simulink model "W03_Pendulum_NonlinVsLin"  (R2024b)
settings: Solver=ode45  StartTime=0.0  StopTime=t_end  MaxStep=0.01  RelTol=1e-3
PreLoadFcn:
  | % W03_Pendulum_NonlinVsLin 기본 파라미터 (모델을 열 때 자동 실행)
  | % 이미 워크스페이스에 값이 있으면 그대로 두고, 없을 때만 채웁니다.
  | defs = { 'm',0.5 ; 'l',0.3 ; 'b',0 ; 'g',9.81 ;
  |          'u_torque',0 ; 'theta0',pi/3 ; 't_end',10 };
  | for ii = 1:size(defs,1)
  |     if ~evalin('base', sprintf('exist(''%s'',''var'')', defs{ii,1}))
  |         assignin('base', defs{ii,1}, defs{ii,2});
  |     end
  | end
  | clear defs ii
values from neighbouring files (symbols this model uses):
  b = 0.2    [W03_02_state_space.m]    (also in W03_04_run_simulink.m = p.b; W03_05_linearize_verify.m = 0.15)
  g = p.g    [W03_04_run_simulink.m]    (also in W03_05_linearize_verify.m = 9.81)
  l = p.l    [W03_04_run_simulink.m]    (also in W03_05_linearize_verify.m = 0.3)
  m = 1    [W03_02_state_space.m]    (also in W03_04_run_simulink.m = p.m; W03_05_linearize_verify.m = 0.5)
  theta0 = deg2rad(angle_list(i))    [W03_04_run_simulink.m]    (also in W03_05_linearize_verify.m = 0)
  u_torque = 0    [W03_04_run_simulink.m]    (also in W03_05_linearize_verify.m)
settings Model: Creator=admin  LastModifiedBy=admin

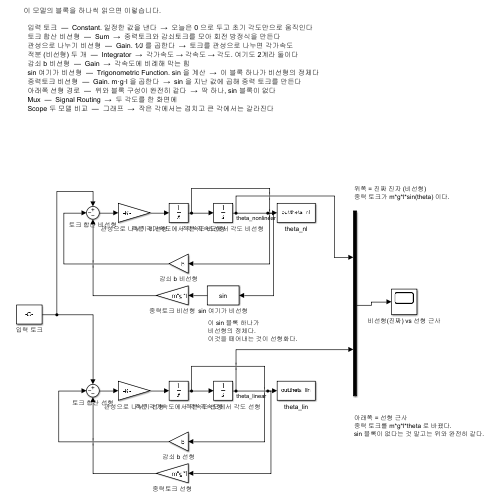
[thumbnail: Simulink's stored preview of the top-level diagram]
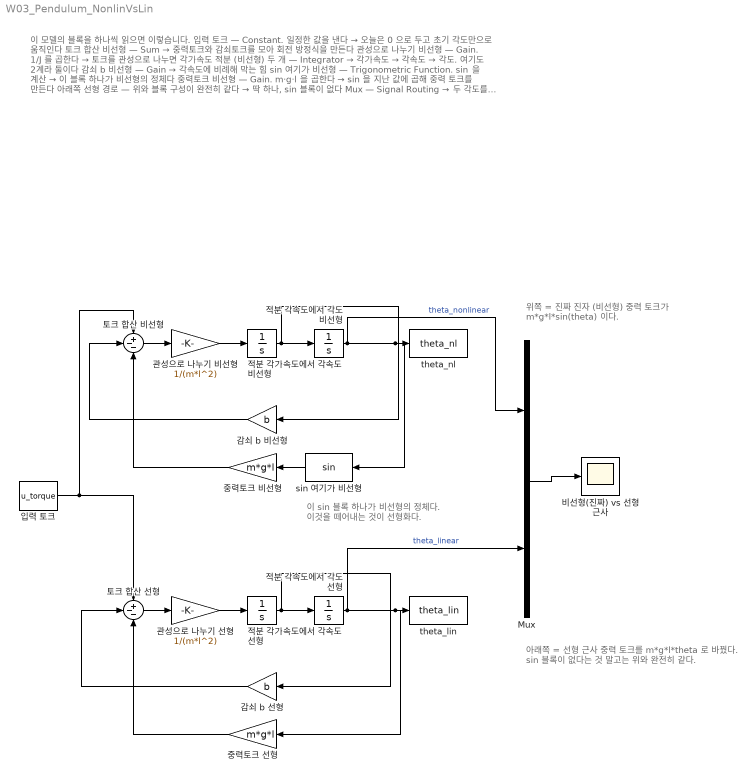
== system W03_Pendulum_NonlinVsLin ==
  note: 위쪽 = 진짜 진자 (비선형)
      | 중력 토크가 m*g*l*sin(theta) 이다.
  note: 아래쪽 = 선형 근사
      | 중력 토크를 m*g*l*theta 로 바꿨다.
      | sin 블록이 없다는 것 말고는 위와 완전히 같다.
  note: 이 sin 블록 하나가
      | 비선형의 정체다.
      | 이것을 떼어내는 것이 선형화다.
  note: 이 모델의 블록을 하나씩 읽으면 이렇습니다.
      |
      |   입력 토크  —  Constant. 일정한 값을 낸다  →  오늘은 0 으로 두고 초기 각도만으로 움직인다
      |   토크 합산 비선형  —  Sum  →  중력토크와 감쇠토크를 모아 회전 방정식을 만든다
      |   관성으로 나누기 비선형  —  Gain. 1∕J 를 곱한다  →  토크를 관성으로 나누면 각가속도
      |   적분 (비선형) 두 개  —  Integrator  →  각가속도 → 각속도 → 각도. 여기도 2계라 둘이다
      |   감쇠 b 비선형  —  Gain  →  각속도에 비례해 막는 힘
      |   sin 여기가 비선형  —  Trigonometric Function. sin 을 계산  →  이 블록 하나가 비선형의 정체다
      |   중력토크 비선형  —  Gain. m·g·l 을 곱한다  →  sin 을 지난 값에 곱해 중력 토크를 만든다
      |   아래쪽 선형 경로  —  위와 블록 구성이 완전히 같다  →  딱 하나, sin 블록이 없다
      |   Mux  —  Signal Routing  →  두 각도를 한 화면에
      |   Scope 두 모델 비교  —  그래프  →  작은 각에서는 겹치고 큰 각에서는 갈라진다
  Mux : Mux  Inputs=2
  sin 여기가 비선형 : Trigonometry
  theta_lin : ToWorkspace  VariableName=theta_lin  SaveFormat=Timeseries  SampleTime=-1
  theta_nl : ToWorkspace  VariableName=theta_nl  SaveFormat=Timeseries  SampleTime=-1
  감쇠 b 비선형 : Gain  Gain=b
  감쇠 b 선형 : Gain  Gain=b
  관성으로 나누기 비선형 : Gain  Gain=1/(m*l^2)
  관성으로 나누기 선형 : Gain  Gain=1/(m*l^2)
  비선형(진짜) vs 선형 근사 : Scope
  입력 토크 : Constant  Value=u_torque
  적분 각가속도에서 각속도 비선형 : Integrator
  적분 각가속도에서 각속도 선형 : Integrator
  적분 각속도에서 각도 비선형 : Integrator  InitialCondition=theta0
  적분 각속도에서 각도 선형 : Integrator  InitialCondition=theta0
  중력토크 비선형 : Gain  Gain=m*g*l
  중력토크 선형 : Gain  Gain=m*g*l
  토크 합산 비선형 : Sum  Inputs=+--
  토크 합산 선형 : Sum  Inputs=+--
  wires:
  입력 토크/1 -> 토크 합산 비선형/1, 토크 합산 선형/1
  토크 합산 비선형/1 -> 관성으로 나누기 비선형/1
  관성으로 나누기 비선형/1 -> 적분 각가속도에서 각속도 비선형/1
  적분 각가속도에서 각속도 비선형/1 -> 적분 각속도에서 각도 비선형/1, 감쇠 b 비선형/1
  감쇠 b 비선형/1 -> 토크 합산 비선형/2
  적분 각속도에서 각도 비선형/1 -> sin 여기가 비선형/1, theta_nl/1, Mux/1  "theta_nonlinear"
  sin 여기가 비선형/1 -> 중력토크 비선형/1
  중력토크 비선형/1 -> 토크 합산 비선형/3
  토크 합산 선형/1 -> 관성으로 나누기 선형/1
  관성으로 나누기 선형/1 -> 적분 각가속도에서 각속도 선형/1
  적분 각가속도에서 각속도 선형/1 -> 적분 각속도에서 각도 선형/1, 감쇠 b 선형/1
  감쇠 b 선형/1 -> 토크 합산 선형/2
  적분 각속도에서 각도 선형/1 -> 중력토크 선형/1, theta_lin/1, Mux/2  "theta_linear"
  중력토크 선형/1 -> 토크 합산 선형/3
  Mux/1 -> 비선형(진짜) vs 선형 근사/1
